simulink model "PID"  (R2021a)
settings: Solver=ode45  StartTime=0.0  StopTime=4  RelTol=1e-3
undefined symbols (not defined in the file): AW, daq, drv, est_par, gbox, mld, mot, PID, rads2rpm, sens
settings Model: Creator=gioel  LastModifiedBy=gioel
settings SolverCC: AlgebraicLoopSolver=TrustRegion
settings DataIOCC: ReturnWorkspaceOutputs=off
settings DebuggingCC: SFMachineParentedDataDiag=warning

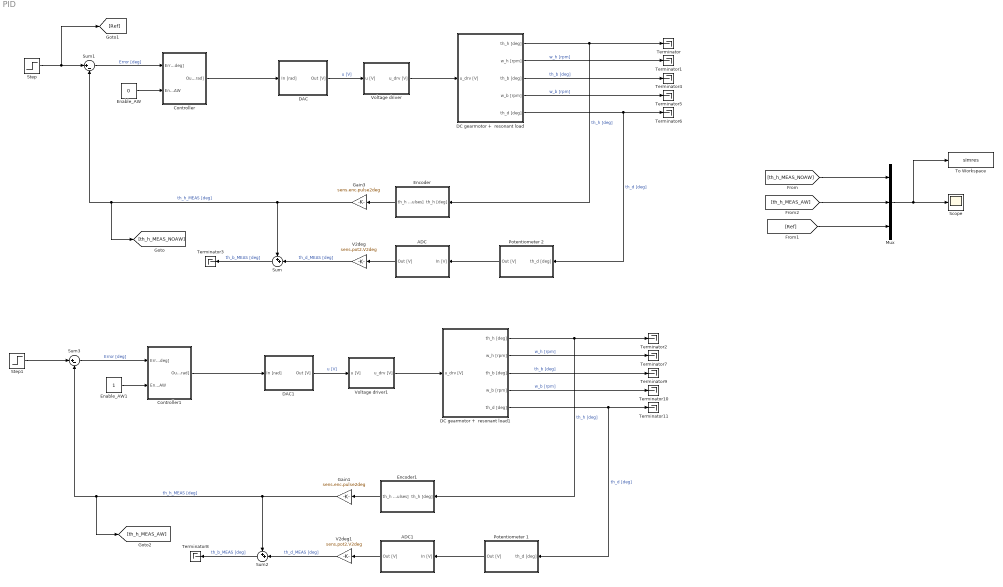
== system PID ==
  ADC : Subsystem
  ADC1 : Subsystem
  Controller : Subsystem
  Controller1 : Subsystem
  DAC : Subsystem
  DAC1 : Subsystem
  DC gearmotor +  resonant load : Subsystem
  DC gearmotor +  resonant load1 : Subsystem
  Enable_AW : Constant  Value=0
  Enable_AW1 : Constant
  Encoder : Subsystem
  Encoder1 : Subsystem
  Gain1 : Gain  Gain=sens.enc.pulse2deg
  Gain3 : Gain  Gain=sens.enc.pulse2deg
  Mux : Mux  Inputs=3
  Potentiometer 1 : Subsystem
  Potentiometer 2 : Subsystem
  Scope : Scope
  Step : Step  Time=0  After=120  SampleTime=0
  Step1 : Step  Time=0  After=120  SampleTime=0
  Sum : Sum  Inputs=++|
  Sum1 : Sum  Inputs=|+-
  Sum2 : Sum  Inputs=++|
  Sum3 : Sum  Inputs=|+-
  Terminator{,1..11} (12 alike) : Terminator
  To Workspace : ToWorkspace  VariableName=simres  SaveFormat=Structure With Time  SampleTime=-1
  V2deg : Gain  Gain=sens.pot2.V2deg
  V2deg1 : Gain  Gain=sens.pot2.V2deg
  Voltage driver : Subsystem
  Voltage driver1 : Subsystem
  wires:
  DAC/1(Out [V]) -> Voltage driver/1(u [V])  "u [V]"
  Encoder/1(th_h [pulses]) -> Gain3/1
  Controller/1(Out [rad]) -> DAC/1(In [rad])
  Potentiometer 2/1(Out [V]) -> ADC/1(In [V])
  ADC/1(Out [V]) -> V2deg/1
  V2deg/1 -> Sum/2  "th_d_MEAS [deg]"
  Gain3/1 -> Sum1/2, [th_h_MEAS_NOAW], Sum/1  "th_h_MEAS [deg]"
  Sum/1 -> Terminator3/1  "th_b_MEAS [deg]"
  Voltage driver/1(u_drv [V]) -> DC gearmotor +  resonant load/1(u_drv [V])
  DC gearmotor +  resonant load/1(th_h [deg]) -> Terminator/1, Encoder/1(th_h [deg])  "th_h [deg]"
  DC gearmotor +  resonant load/2(w_h [rpm]) -> Terminator1/1  "w_h [rpm]"
  DC gearmotor +  resonant load/3(th_b [deg]) -> Terminator4/1  "th_b [deg]"
  DC gearmotor +  resonant load/4(w_b [rpm]) -> Terminator5/1  "w_b [rpm]"
  DC gearmotor +  resonant load/5(th_d [deg]) -> Terminator6/1, Potentiometer 2/1(th_d [deg])  "th_d [deg]"
  Sum1/1 -> Controller/1(Error [deg])  "Error [deg]"
  Step/1 -> [Ref], Sum1/1
  Enable_AW/1 -> Controller/2(Enable_AW)
  Mux/1 -> To Workspace/1, Scope/1
  [th_h_MEAS_NOAW] -> Mux/1
  Enable_AW1/1 -> Controller1/2(Enable_AW)
  Step1/1 -> Sum3/1
  Sum3/1 -> Controller1/1(Error [deg])  "Error [deg]"
  DC gearmotor +  resonant load1/5(th_d [deg]) -> Potentiometer 1/1(th_d [deg]), Terminator11/1  "th_d [deg]"
  DC gearmotor +  resonant load1/4(w_b [rpm]) -> Terminator10/1  "w_b [rpm]"
  DC gearmotor +  resonant load1/3(th_b [deg]) -> Terminator9/1  "th_b [deg]"
  DC gearmotor +  resonant load1/2(w_h [rpm]) -> Terminator7/1  "w_h [rpm]"
  DC gearmotor +  resonant load1/1(th_h [deg]) -> Encoder1/1(th_h [deg]), Terminator2/1  "th_h [deg]"
  Voltage driver1/1(u_drv [V]) -> DC gearmotor +  resonant load1/1(u_drv [V])
  Sum2/1 -> Terminator8/1  "th_b_MEAS [deg]"
  Gain1/1 -> Sum2/1, [th_h_MEAS_AW], Sum3/2  "th_h_MEAS [deg]"
  V2deg1/1 -> Sum2/2  "th_d_MEAS [deg]"
  ADC1/1(Out [V]) -> V2deg1/1
  Potentiometer 1/1(Out [V]) -> ADC1/1(In [V])
  Controller1/1(Out [rad]) -> DAC1/1(In [rad])
  Encoder1/1(th_h [pulses]) -> Gain1/1
  DAC1/1(Out [V]) -> Voltage driver1/1(u [V])  "u [V]"
  [Ref] -> Mux/3
  [th_h_MEAS_AW] -> Mux/2

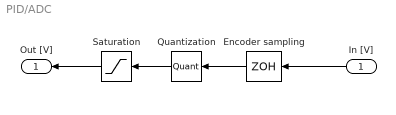
== system PID/ADC ==
  In [V] : Inport
  Encoder sampling : ZeroOrderHold  SampleTime=sens.enc.T_s
  Quantization : Quantizer  QuantizationInterval=daq.adc.q
  Saturation : Saturate  UpperLimit=daq.adc.fs  LowerLimit=-daq.adc.fs
  Out [V] : Outport
  wires:
  Encoder sampling/1 -> Quantization/1
  Quantization/1 -> Saturation/1
  In [V]/1 -> Encoder sampling/1
  Saturation/1 -> Out [V]/1

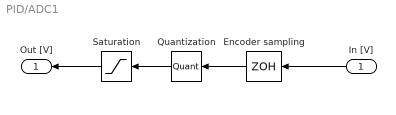
== system PID/ADC1 ==
  In [V] : Inport
  Encoder sampling : ZeroOrderHold  SampleTime=sens.enc.T_s
  Quantization : Quantizer  QuantizationInterval=daq.adc.q
  Saturation : Saturate  UpperLimit=daq.adc.fs  LowerLimit=-daq.adc.fs
  Out [V] : Outport
  wires:
  Saturation/1 -> Out [V]/1
  In [V]/1 -> Encoder sampling/1
  Quantization/1 -> Saturation/1
  Encoder sampling/1 -> Quantization/1

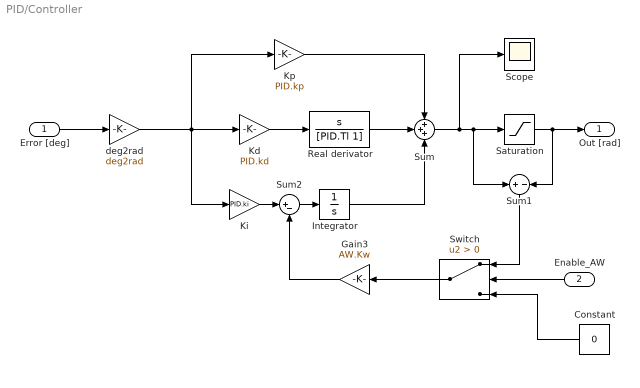
== system PID/Controller ==
  Error [deg] : Inport
  Enable_AW : Inport  Port=2
  Constant : Constant  Value=0
  Gain3 : Gain  Gain=AW.Kw
  Integrator : Integrator
  Kd : Gain  Gain=PID.kd
  Ki : Gain  Gain=PID.ki
  Kp : Gain  Gain=PID.kp
  Real derivator : TransferFcn  Numerator=[1 0]  Denominator=[PID.Tl 1]
  Saturation : Saturate  UpperLimit=10  LowerLimit=-10
  Scope : Scope
  Sum : Sum  Inputs=+++
  Sum1 : Sum  Inputs=+-
  Sum2 : Sum  Inputs=|+-
  Switch : Switch  Criteria=u2 > Threshold
  deg2rad : Gain  Gain=deg2rad
  Out [rad] : Outport
  wires:
  Real derivator/1 -> Sum/2
  Integrator/1 -> Sum/3
  Kp/1 -> Sum/1
  Kd/1 -> Real derivator/1
  Sum/1 -> Scope/1, Sum1/1, Saturation/1
  Saturation/1 -> Sum1/2, Out [rad]/1
  Sum1/1 -> Switch/1
  Switch/1 -> Gain3/1
  Gain3/1 -> Sum2/2
  Ki/1 -> Sum2/1
  Sum2/1 -> Integrator/1
  Enable_AW/1 -> Switch/2
  Constant/1 -> Switch/3
  Error [deg]/1 -> deg2rad/1
  deg2rad/1 -> Ki/1, Kp/1, Kd/1

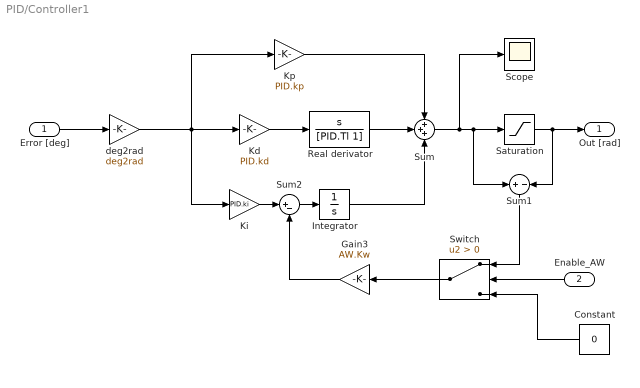
== system PID/Controller1 ==
  Error [deg] : Inport
  Enable_AW : Inport  Port=2
  Constant : Constant  Value=0
  Gain3 : Gain  Gain=AW.Kw
  Integrator : Integrator
  Kd : Gain  Gain=PID.kd
  Ki : Gain  Gain=PID.ki
  Kp : Gain  Gain=PID.kp
  Real derivator : TransferFcn  Numerator=[1 0]  Denominator=[PID.Tl 1]
  Saturation : Saturate  UpperLimit=10  LowerLimit=-10
  Scope : Scope
  Sum : Sum  Inputs=+++
  Sum1 : Sum  Inputs=+-
  Sum2 : Sum  Inputs=|+-
  Switch : Switch  Criteria=u2 > Threshold
  deg2rad : Gain  Gain=deg2rad
  Out [rad] : Outport
  wires:
  deg2rad/1 -> Kd/1, Kp/1, Ki/1
  Error [deg]/1 -> deg2rad/1
  Constant/1 -> Switch/3
  Enable_AW/1 -> Switch/2
  Sum2/1 -> Integrator/1
  Ki/1 -> Sum2/1
  Gain3/1 -> Sum2/2
  Switch/1 -> Gain3/1
  Sum1/1 -> Switch/1
  Saturation/1 -> Out [rad]/1, Sum1/2
  Sum/1 -> Saturation/1, Sum1/1, Scope/1
  Kd/1 -> Real derivator/1
  Kp/1 -> Sum/1
  Integrator/1 -> Sum/3
  Real derivator/1 -> Sum/2

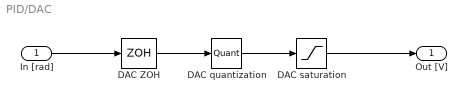
== system PID/DAC ==
  In [rad] : Inport
  DAC ZOH : ZeroOrderHold  SampleTime=sens.enc.T_s
  DAC quantization : Quantizer  QuantizationInterval=daq.dac.q
  DAC saturation : Saturate  UpperLimit=daq.dac.vdd  LowerLimit=daq.dac.vss
  Out [V] : Outport
  wires:
  DAC quantization/1 -> DAC saturation/1
  DAC ZOH/1 -> DAC quantization/1
  DAC saturation/1 -> Out [V]/1
  In [rad]/1 -> DAC ZOH/1

== system PID/DAC1 ==
  In [rad] : Inport
  DAC ZOH : ZeroOrderHold  SampleTime=sens.enc.T_s
  DAC quantization : Quantizer  QuantizationInterval=daq.dac.q
  DAC saturation : Saturate  UpperLimit=daq.dac.vdd  LowerLimit=daq.dac.vss
  Out [V] : Outport
  wires:
  In [rad]/1 -> DAC ZOH/1
  DAC saturation/1 -> Out [V]/1
  DAC ZOH/1 -> DAC quantization/1
  DAC quantization/1 -> DAC saturation/1

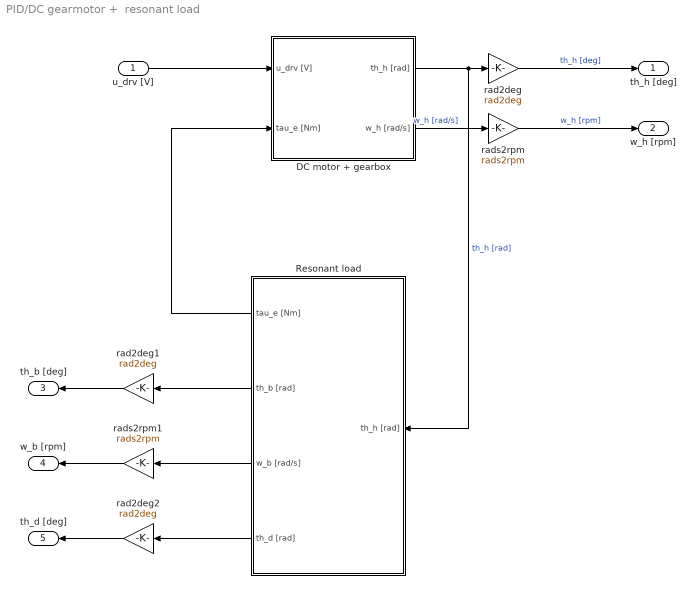
== system PID/DC gearmotor +  resonant load ==
  u_drv [V] : Inport
  DC motor + gearbox : Subsystem
  Resonant load : Subsystem
  rad2deg : Gain  Gain=rad2deg
  rad2deg1 : Gain  Gain=rad2deg
  rad2deg2 : Gain  Gain=rad2deg
  rads2rpm : Gain  Gain=rads2rpm
  rads2rpm1 : Gain  Gain=rads2rpm
  th_h [deg] : Outport
  w_h [rpm] : Outport  Port=2
  th_b [deg] : Outport  Port=3
  w_b [rpm] : Outport  Port=4
  th_d [deg] : Outport  Port=5
  wires:
  rads2rpm1/1 -> w_b [rpm]/1
  Resonant load/1(tau_e [Nm]) -> DC motor + gearbox/2(tau_e [Nm])
  DC motor + gearbox/2(w_h [rad/s]) -> rads2rpm/1  "w_h [rad/s]"
  rad2deg1/1 -> th_b [deg]/1
  u_drv [V]/1 -> DC motor + gearbox/1(u_drv [V])
  Resonant load/3(w_b [rad/s]) -> rads2rpm1/1
  rad2deg2/1 -> th_d [deg]/1
  Resonant load/4(th_d [rad]) -> rad2deg2/1
  Resonant load/2(th_b [rad]) -> rad2deg1/1
  rad2deg/1 -> th_h [deg]/1  "th_h [deg]"
  rads2rpm/1 -> w_h [rpm]/1  "w_h [rpm]"
  DC motor + gearbox/1(th_h [rad]) -> Resonant load/1(th_h [rad]), rad2deg/1  "th_h [rad]"

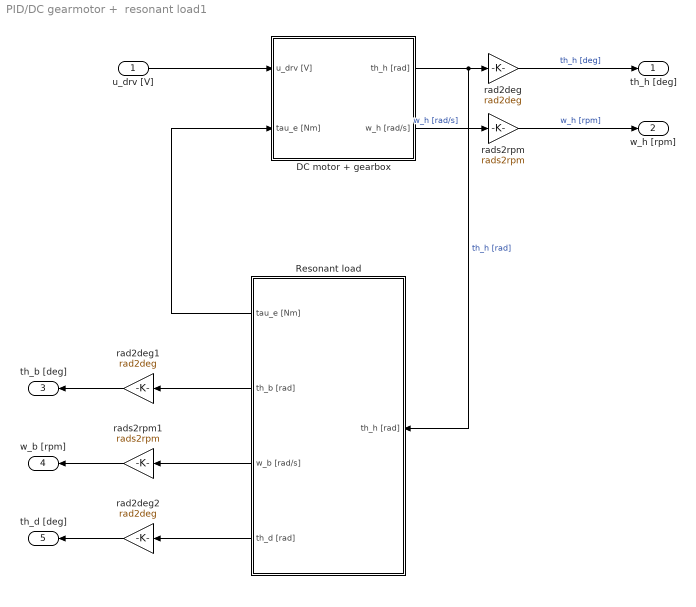
== system PID/DC gearmotor +  resonant load1 ==
  u_drv [V] : Inport
  DC motor + gearbox : Subsystem
  Resonant load : Subsystem
  rad2deg : Gain  Gain=rad2deg
  rad2deg1 : Gain  Gain=rad2deg
  rad2deg2 : Gain  Gain=rad2deg
  rads2rpm : Gain  Gain=rads2rpm
  rads2rpm1 : Gain  Gain=rads2rpm
  th_h [deg] : Outport
  w_h [rpm] : Outport  Port=2
  th_b [deg] : Outport  Port=3
  w_b [rpm] : Outport  Port=4
  th_d [deg] : Outport  Port=5
  wires:
  DC motor + gearbox/1(th_h [rad]) -> rad2deg/1, Resonant load/1(th_h [rad])  "th_h [rad]"
  rads2rpm/1 -> w_h [rpm]/1  "w_h [rpm]"
  rad2deg/1 -> th_h [deg]/1  "th_h [deg]"
  Resonant load/2(th_b [rad]) -> rad2deg1/1
  Resonant load/4(th_d [rad]) -> rad2deg2/1
  rad2deg2/1 -> th_d [deg]/1
  Resonant load/3(w_b [rad/s]) -> rads2rpm1/1
  u_drv [V]/1 -> DC motor + gearbox/1(u_drv [V])
  rad2deg1/1 -> th_b [deg]/1
  DC motor + gearbox/2(w_h [rad/s]) -> rads2rpm/1  "w_h [rad/s]"
  Resonant load/1(tau_e [Nm]) -> DC motor + gearbox/2(tau_e [Nm])
  rads2rpm1/1 -> w_b [rpm]/1

== system PID/Encoder ==
  th_h [deg] : Inport
  Deg2pulse : Gain  Gain=sens.enc.deg2pulse
  Encoder sampling : ZeroOrderHold  SampleTime=sens.enc.T_s
  Quantization : Quantizer  QuantizationInterval=sens.enc.q
  th_h [pulses] : Outport
  wires:
  Encoder sampling/1 -> Quantization/1
  Quantization/1 -> Deg2pulse/1
  th_h [deg]/1 -> Encoder sampling/1
  Deg2pulse/1 -> th_h [pulses]/1

== system PID/Encoder1 ==
  th_h [deg] : Inport
  Deg2pulse : Gain  Gain=sens.enc.deg2pulse
  Encoder sampling : ZeroOrderHold  SampleTime=sens.enc.T_s
  Quantization : Quantizer  QuantizationInterval=sens.enc.q
  th_h [pulses] : Outport
  wires:
  Deg2pulse/1 -> th_h [pulses]/1
  th_h [deg]/1 -> Encoder sampling/1
  Quantization/1 -> Deg2pulse/1
  Encoder sampling/1 -> Quantization/1

== system PID/Potentiometer 1 ==
  th_d [deg] : Inport
  Sensor output noise [V] : RandomNumber  Variance=sens.pot2.noise.var  SampleTime=0.1
  Sum : Sum  Inputs=++|
  deg2V : Gain  Gain=sens.pot2.deg2V
  Out [V] : Outport
  wires:
  Sensor output noise [V]/1 -> Sum/1
  deg2V/1 -> Sum/2
  th_d [deg]/1 -> deg2V/1
  Sum/1 -> Out [V]/1

== system PID/Potentiometer 2 ==
  th_d [deg] : Inport
  Sensor output noise [V] : RandomNumber  Variance=sens.pot2.noise.var  SampleTime=0.1
  Sum : Sum  Inputs=++|
  deg2V : Gain  Gain=sens.pot2.deg2V
  Out [V] : Outport
  wires:
  Sum/1 -> Out [V]/1
  th_d [deg]/1 -> deg2V/1
  deg2V/1 -> Sum/2
  Sensor output noise [V]/1 -> Sum/1

== system PID/Voltage driver ==
  u [V] : Inport
  Driver dynamics : TransferFcn  Numerator=[drv.dcgain]  Denominator=[drv.Tc 1]
  Driver saturation : Saturate  UpperLimit=drv.outmax  LowerLimit=-drv.outmax
  u_drv [V] : Outport
  wires:
  Driver saturation/1 -> u_drv [V]/1
  Driver dynamics/1 -> Driver saturation/1
  u [V]/1 -> Driver dynamics/1

== system PID/Voltage driver1 ==
  u [V] : Inport
  Driver dynamics : TransferFcn  Numerator=[drv.dcgain]  Denominator=[drv.Tc 1]
  Driver saturation : Saturate  UpperLimit=drv.outmax  LowerLimit=-drv.outmax
  u_drv [V] : Outport
  wires:
  u [V]/1 -> Driver dynamics/1
  Driver dynamics/1 -> Driver saturation/1
  Driver saturation/1 -> u_drv [V]/1

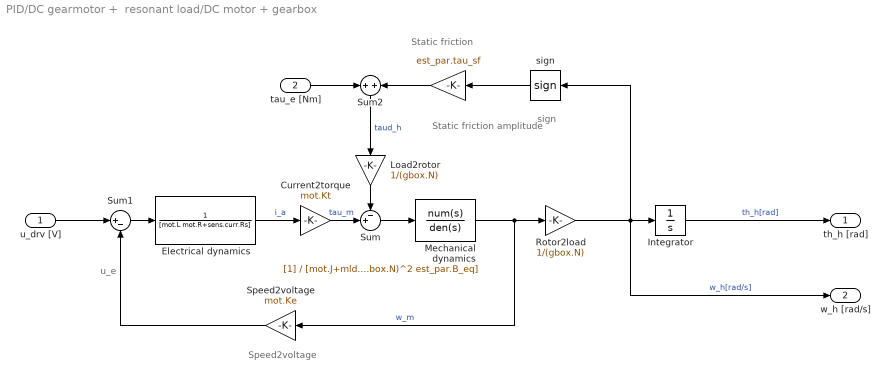
== system PID/DC gearmotor +  resonant load/DC motor + gearbox ==
  note: u_e
  note: Speed2voltage
  note: Static friction
  note: sign
  note: Static friction
      |  amplitude
  u_drv [V] : Inport
  tau_e [Nm] : Inport  Port=2
  " " : Gain  Gain=est_par.tau_sf
  Current2torque : Gain  Gain=mot.Kt
  Electrical dynamics : TransferFcn  Denominator=[mot.L mot.R+sens.curr.Rs]
  Integrator : Integrator
  Load2rotor : Gain  Gain=1/(gbox.N)
  Mechanical dynamics : TransferFcn  Denominator=[mot.J+mld.Jh/(gbox.N)^2 est_par.B_eq]
  Rotor2load : Gain  Gain=1/(gbox.N)
  Speed2voltage : Gain  Gain=mot.Ke
  Sum : Sum  Inputs=-+|
  Sum1 : Sum  Inputs=|+-
  Sum2 : Sum  Inputs=+|+
  sign : Signum  ZeroCross=off
  th_h [rad] : Outport
  w_h [rad/s] : Outport  Port=2
  wires:
  u_drv [V]/1 -> Sum1/1
  Electrical dynamics/1 -> Current2torque/1  "i_a"
  Current2torque/1 -> Sum/2  "tau_m"
  sign/1 -> " "/1
  Sum1/1 -> Electrical dynamics/1
  Integrator/1 -> th_h [rad]/1  "th_h[rad]"
  Sum/1 -> Mechanical dynamics/1
  Load2rotor/1 -> Sum/1
  Speed2voltage/1 -> Sum1/2
  Rotor2load/1 -> w_h [rad/s]/1, sign/1, Integrator/1  "w_h[rad/s]"
  Mechanical dynamics/1 -> Speed2voltage/1, Rotor2load/1  "w_m"
  " "/1 -> Sum2/2
  Sum2/1 -> Load2rotor/1  "taud_h"
  tau_e [Nm]/1 -> Sum2/1

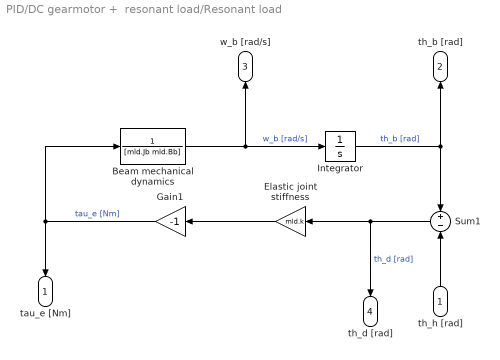
== system PID/DC gearmotor +  resonant load/Resonant load ==
  th_h [rad] : Inport
  Beam mechanical dynamics : TransferFcn  Denominator=[mld.Jb mld.Bb]
  Elastic joint stiffness : Gain  Gain=mld.k
  Gain1 : Gain  Gain=-1
  Integrator : Integrator
  Sum1 : Sum  Inputs=+|-
  tau_e [Nm] : Outport
  th_b [rad] : Outport  Port=2
  w_b [rad/s] : Outport  Port=3
  th_d [rad] : Outport  Port=4
  wires:
  th_h [rad]/1 -> Sum1/2
  Gain1/1 -> tau_e [Nm]/1, Beam mechanical dynamics/1  "tau_e [Nm]"
  Elastic joint stiffness/1 -> Gain1/1
  Sum1/1 -> th_d [rad]/1, Elastic joint stiffness/1  "th_d [rad]"
  Integrator/1 -> th_b [rad]/1, Sum1/1  "th_b [rad]"
  Beam mechanical dynamics/1 -> w_b [rad/s]/1, Integrator/1  "w_b [rad/s]"

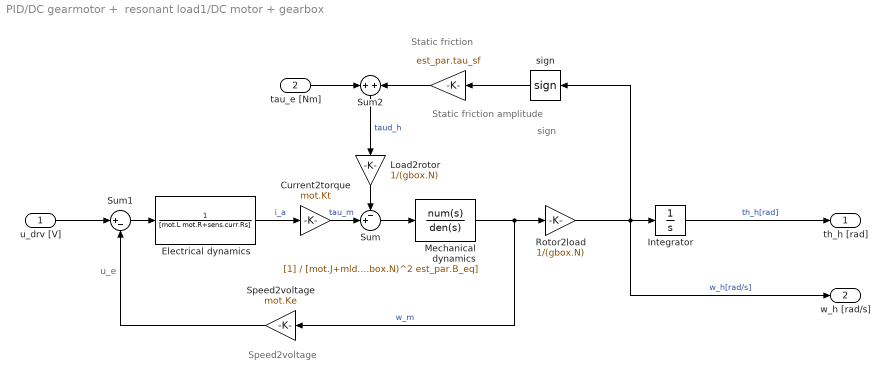
== system PID/DC gearmotor +  resonant load1/DC motor + gearbox ==
  note: Static friction
      |  amplitude
  note: sign
  note: Static friction
  note: Speed2voltage
  note: u_e
  u_drv [V] : Inport
  tau_e [Nm] : Inport  Port=2
  " " : Gain  Gain=est_par.tau_sf
  Current2torque : Gain  Gain=mot.Kt
  Electrical dynamics : TransferFcn  Denominator=[mot.L mot.R+sens.curr.Rs]
  Integrator : Integrator
  Load2rotor : Gain  Gain=1/(gbox.N)
  Mechanical dynamics : TransferFcn  Denominator=[mot.J+mld.Jh/(gbox.N)^2 est_par.B_eq]
  Rotor2load : Gain  Gain=1/(gbox.N)
  Speed2voltage : Gain  Gain=mot.Ke
  Sum : Sum  Inputs=-+|
  Sum1 : Sum  Inputs=|+-
  Sum2 : Sum  Inputs=+|+
  sign : Signum  ZeroCross=off
  th_h [rad] : Outport
  w_h [rad/s] : Outport  Port=2
  wires:
  tau_e [Nm]/1 -> Sum2/1
  Sum2/1 -> Load2rotor/1  "taud_h"
  " "/1 -> Sum2/2
  Mechanical dynamics/1 -> Rotor2load/1, Speed2voltage/1  "w_m"
  Rotor2load/1 -> Integrator/1, sign/1, w_h [rad/s]/1  "w_h[rad/s]"
  Speed2voltage/1 -> Sum1/2
  Load2rotor/1 -> Sum/1
  Sum/1 -> Mechanical dynamics/1
  Integrator/1 -> th_h [rad]/1  "th_h[rad]"
  Sum1/1 -> Electrical dynamics/1
  sign/1 -> " "/1
  Current2torque/1 -> Sum/2  "tau_m"
  Electrical dynamics/1 -> Current2torque/1  "i_a"
  u_drv [V]/1 -> Sum1/1

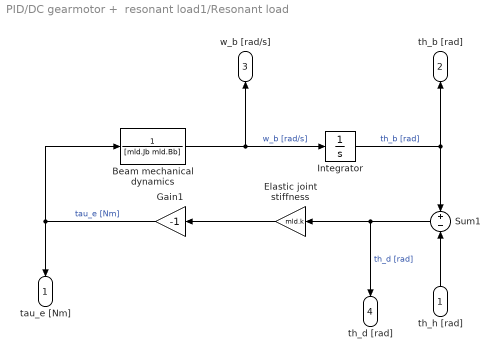
== system PID/DC gearmotor +  resonant load1/Resonant load ==
  th_h [rad] : Inport
  Beam mechanical dynamics : TransferFcn  Denominator=[mld.Jb mld.Bb]
  Elastic joint stiffness : Gain  Gain=mld.k
  Gain1 : Gain  Gain=-1
  Integrator : Integrator
  Sum1 : Sum  Inputs=+|-
  tau_e [Nm] : Outport
  th_b [rad] : Outport  Port=2
  w_b [rad/s] : Outport  Port=3
  th_d [rad] : Outport  Port=4
  wires:
  Beam mechanical dynamics/1 -> Integrator/1, w_b [rad/s]/1  "w_b [rad/s]"
  Integrator/1 -> Sum1/1, th_b [rad]/1  "th_b [rad]"
  Sum1/1 -> Elastic joint stiffness/1, th_d [rad]/1  "th_d [rad]"
  Elastic joint stiffness/1 -> Gain1/1
  Gain1/1 -> Beam mechanical dynamics/1, tau_e [Nm]/1  "tau_e [Nm]"
  th_h [rad]/1 -> Sum1/2
